simulink model "Pipe_TemperatureStep"  (R2013b)
settings: Solver=ode45  StartTime=0.0  StopTime=120  RelTol=1e-5
libraries: carnot x6
settings Model: Creator=drhf  LastModifiedBy=drhf
settings DataIOCC: SignalLoggingSaveFormat=ModelDataLogs
settings OptimizationCC: ExpressionDepthLimit=2147483647
settings DebuggingCC: FcnCallInpInsideContextMsg=UseLocalSettings  StateNameClashWarn=warning
settings GRTTargetCC: CombineOutputUpdateFcns=off  GRTInterface=on

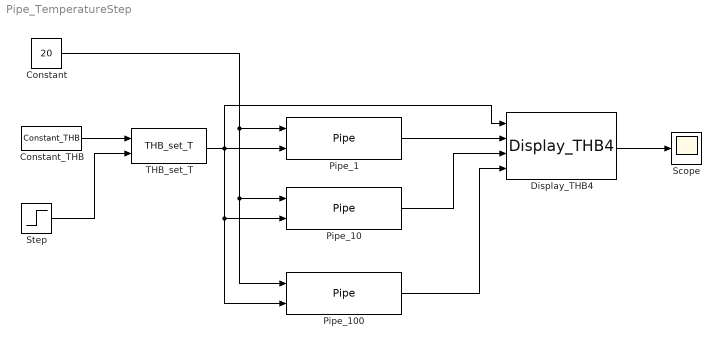
== system Pipe_TemperatureStep ==
  Constant : Constant  Value=20
  Constant_THB : carnot/Source/Simple/Constant_THB  t=40  mdot=0.21  p=3e5  mID=No Pressure Drop  fluid=Water  mix=0  mix2=0  mix3=0  dia=10  hgt=0
  Display_THB4 : carnot/Outputs/Display_THB4  t=on  m=off  p=off  id=off  mix=off  d=off
  Pipe_1 : carnot/Hydraulics/Pipe  dia=0.027  len=10  hgt=0  uloss=0  cond=0  cwall=1000  t0=20  lin=100/0.2  qua=100/0.2^2  nodes=1
  Pipe_10 : carnot/Hydraulics/Pipe  dia=0.027  len=10  hgt=0  uloss=0  cond=0  cwall=1000  t0=20  lin=100/0.2  qua=100/0.2^2  nodes=10
  Pipe_100 : carnot/Hydraulics/Pipe  dia=0.027  len=10  hgt=0  uloss=0  cond=0  cwall=1000  t0=20  lin=100/0.2  qua=100/0.2^2  nodes=100
  Scope : Scope
      settings: TimeRange=4000  YMin=39.66951326595616  YMax=40.42277164649369
  Step : Step  Time=10  Before=20  After=60  SampleTime=0
  THB_set_T : carnot/Source/Simple/THB_set_T
  wires:
  Constant/1 -> Pipe_10/1, Pipe_100/1, Pipe_1/1
  Pipe_1/1 -> Display_THB4/2
  Constant_THB/1 -> THB_set_T/1
  THB_set_T/1 -> Pipe_100/2, Pipe_10/2, Display_THB4/1, Pipe_1/2
  Display_THB4/1 -> Scope/1
  Step/1 -> THB_set_T/2
  Pipe_10/1 -> Display_THB4/3
  Pipe_100/1 -> Display_THB4/4
